simulink model "design_firfilter"  (R2015a)
settings: Solver=ode45  StartTime=0.0  StopTime=20  RelTol=1e-3
libraries: simulink x1
settings Model: Creator=liuqi  LastModifiedBy=liuqi

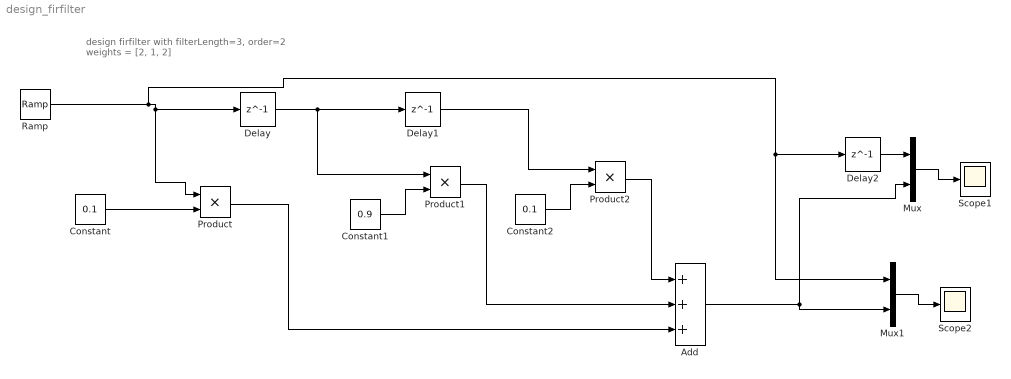
== system design_firfilter ==
  note: design firfilter with filterLength=3, order=2
      | weights = [2, 1, 2]
  Add : Sum  Inputs=+++
  Constant : Constant  Value=0.1
  Constant1 : Constant  Value=0.9
  Constant2 : Constant  Value=0.1
  Delay : Delay  DelayLength=1  InitialCondition=0  SampleTime=1
  Delay1 : Delay  DelayLength=1  InitialCondition=0
  Delay2 : Delay  DelayLength=1  InitialCondition=0  SampleTime=1
  Mux : Mux  Inputs=2
  Mux1 : Mux  Inputs=2
  Product : Product
  Product1 : Product
  Product2 : Product
  Ramp : simulink/Sources/Ramp  slope=1  start=0  X0=0
  Scope1 : Scope
  Scope2 : Scope
  wires:
  Delay/1 -> Product1/1, Delay1/1
  Delay1/1 -> Product2/1
  Constant/1 -> Product/2
  Ramp/1 -> Mux1/1, Delay2/1, Delay/1, Product/1
  Constant1/1 -> Product1/2
  Constant2/1 -> Product2/2
  Product2/1 -> Add/1
  Product1/1 -> Add/2
  Product/1 -> Add/3
  Add/1 -> Mux1/2, Mux/2
  Mux/1 -> Scope1/1
  Delay2/1 -> Mux/1
  Mux1/1 -> Scope2/1
